simulink model "TailSitter_waypoints_continuous"  (R2018b)
settings: Solver=VariableStepAuto  StartTime=0.0  StopTime=400  RelTol=1e-3
values from neighbouring files (symbols this model uses):
  p =     [ds.mat]    (also in vxs.mat)
undefined symbols (not defined in the file or in its folder): quatnormalize
libraries: aerolibutil x18, simulink x6, sharedutil x3, vrlib x2, simulink_extras x2, sharedtransform x1
(part 4 of 4)

== matlab function TailSitter_waypoints_continuous/TailSitter/tailsittersimv2 ==
  data: omegaLdot output; omegaRdot output; deltaLdot output; deltaRdot output; qdot output; wdot output; vdot output; omegaL input; omegaR input; deltaL input; deltaR input; u_omegaL input; u_omegaR input; u_deltaL input; u_deltaR input; q input; w input; v input; p parameter; alpha output; Beta output; g_out output
function [ omegaLdot, omegaRdot, deltaLdot, deltaRdot, qdot,wdot,vdot, alpha, Beta, g_out] = ...
    tailsitter_v2(omegaL, omegaR, deltaL, deltaR, u_omegaL, u_omegaR, u_deltaL, ...
    u_deltaR, q,w,v, p)

% Set output port dim
omegaLdot = 0;
omegaRdot = 0;
deltaLdot = 0;
deltaRdot = 0;
alpha = 0;
Beta = 0;
qdot = zeros(4,1);
wdot = zeros(3,1);
vdot = zeros(3,1);
g_out = zeros(3,1);

% Map inputs
vx = v(1);
vy = v(2);
vz = v(3);

wx = w(1);
wy = w(2);
wz = w(3);

q0 = q(1);
q1 = q(2);
q2 = q(3);
q3 = q(4);

% function handles not supported, so adding here directly
c = @(y) 0.28 - (0.28-0.09).*abs(y)./(p.b/2); % This should be pretty accurate
% Lift curves
CL = @(alpha) p.CL_A*sin(p.CL_B.*alpha)+p.CL_C; % These are wrong, just placeholders
CD = @(alpha) p.CD_A-p.CD_A.*cos(p.CD_B.*alpha)+p.CD_C;

alpha = atan2(vz,vx);

%Thrust
TL = p.K_T .* omegaL.^2;
TR = p.K_T .* omegaR.^2;

% airflow in thrust wake
v_w_L = p.b_w .* omegaL; %[b_w .* omegaL; vy; vz];
v_w_R = p.b_w .* omegaR;
%alpha_wL = atan2(vz,v_w_L);
%alpha_wR = atan2(vz,v_w_R);

% Quaternion
qdot = 0.5.*[-q1 -q2 -q3; ...
            q0 -q3 q2; ...
            q3 q0 -q1; ...
            -q2 q1 q0]*w;

% inputs
deltaLdot = p.K_deltaL .* (-deltaL + u_deltaL);
deltaRdot = p.K_deltaR .* (-deltaR + u_deltaR);
omegaLdot = p.K_omegaL .* (-omegaL + u_omegaL);
omegaRdot = p.K_omegaR .* (-omegaR + u_omegaR);

% gravity
% To get vector g in bf from wf
% we need to rotate it by q_wf, or conj(q_bf)
qc = quatconj([q0 q1 q2 q3]); %
qc0 = qc(1);
qc1 = qc(2);
qc2 = qc(3);
qc3 = qc(4);
gravity = p.g .* [2.*(qc1.*qc3 + qc0.*qc2); ...
                2.*(qc2.*qc3 - qc0.*qc1); ...
                (qc0.^2 - qc1.^2 - qc2.^2 + qc3.^2);
                zeros(3+4+4,1)];
g_out = gravity(1:3,1);
% Inertial forces
inertialF = -[2*(vz.*wy - vy.*wz); ...
             2*(vx.*wz - vz.*wx); ...
             2*(vy.*wx - vx.*wy); ...
             (p.Iz - p.Iy).*wy.*wz./p.Ix; ...
             (p.Ix - p.Iz).*wx.*wz./p.Iy; ...
             (p.Iy - p.Ix).*wx.*wy./p.Iz; ...
             zeros(8,1)];
%Sideslip
Beta = atan2(vy,vx);

% Winglets
CLB = @(beta) p.CLB_A*sin(p.CLB_B.*beta); % These are wrong, just placeholders
CDB = @(beta) p.CDB_A-p.CDB_A.*cos(p.CDB_B.*beta);
L_W = -p.rho * sqrt(vx.^2+vy.^2) * p.SW * (CLB(Beta)*vx + CDB(Beta)*vy); % Lift in bodyframe, y
D_W = p.rho * sqrt(vx.^2+vy.^2) * p.SW * (-CLB(Beta)*vy + CDB(Beta)*vx); % Drag in bodyfram, x

% MAIN WING
% Lift inside wake
LLT = p.Sw_w * 0.5 * p.rho * abs(v_w_L) .* CL(0).*v_w_L ;
LRT = p.Sw_w * 0.5 * p.rho * abs(v_w_R) .* CL(0).*v_w_R ;
% Lift outside wake
LL = p.Sw * 0.5 * p.rho * sqrt(vx.^2 + vz.^2) .* ...
    (CL(alpha).*vx + CD(alpha).*vz);
LR = LL; % Yeah we -could- combine these, but too late!
% Drag inside wake
DLT = p.Sw_w * 0.5 * p.rho * abs(v_w_L) * CD(0) * v_w_L;
DRT = p.Sw_w * 0.5 * p.rho * abs(v_w_R) * CD(0) * v_w_R;
% Drag outside wake
DL = p.Sw * 0.5 * p.rho * sqrt(vx.^2  + vz.^2) .* ...
    (-CL(alpha).*vz + CD(alpha).*vx);
DR = DL; % Yeah, we -could- combine these as well...

% AILERONS
% Lift inside wake, signs bc rotation dir of aileron
FLT = -p.CLdelta * 0.5*p.rho*v_w_L.^2 * p.Saw * deltaL;
FRT = -p.CLdelta * 0.5*p.rho*v_w_R.^2 * p.Saw * deltaR;
% Lift outside wake
FL = -sign(vx).*p.CLdelta * 0.5*p.rho*(vx.^2 + vy.^2 + vz.^2) * p.Sa * deltaL;
FR = -sign(vx).*p.CLdelta * 0.5*p.rho*(vx.^2 + vy.^2 + vz.^2) * p.Sa * deltaR;
% Drag inside wake
DalphaLT =p.CDdelta * 0.5*p.rho*v_w_L.^2 * p.Saw * abs(deltaL);
DalphaRT = p.CDdelta * 0.5*p.rho*v_w_R.^2 * p.Saw * abs(deltaR);
% Drag outside wake, we add sign of vx because we might be reversing?
DalphaL = sign(vx).*p.CDdelta * 0.5*p.rho*(vx.^2 + vy.^2 + vz.^2) * p.Sa * abs(deltaL);
DalphaR = sign(vx).*p.CDdelta * 0.5*p.rho*(vx.^2 + vy.^2 + vz.^2) * p.Sa * abs(deltaR);

% f1
 % diff in ail deflection
  % inside wake
  % outside wake
 % resmom roll,
 % roll due to yaw rate
 % moment due to sideslip
alphal_rmr = @(y) atan2(vz+wx.*y, vx);
restmomroll = @(y) y .* c(y) .* sqrt(vx.^2 + (vz+wx.*y).^2) .* ...
    (CL(alphal_rmr(y)).*vx + CD(alphal_rmr(y)).*(vz+wx.*y));
alphal_rwz = @(y) atan2(vz, vx-wz.*y);
rollduetowz = @(y) y .* c(y) .* sqrt((vx-wz.*y).^2 + vz.^2) .* ...
    (CL(alphal_rwz(y)).*(vx-wz*y) + CD(alphal_rwz(y)).*vz);
f1 = p.yf.*(FLT+FL -FRT-FR) ...
    -0.5*p.rho.*quadgk(restmomroll,-p.yW,p.yW) ... % between wakes
     -0.5*p.rho.*quadgk(restmomroll,-p.yWEE,-p.yWE) ... % outside left wake
      -0.5*p.rho.*quadgk(restmomroll,p.yWE,p.yWEE) ... % outside right wake
    -0.5*p.rho.*quadgk(rollduetowz,-p.yW,p.yW) ... between wakes
     -0.5*p.rho.*quadgk(rollduetowz,-p.yWEE,-p.yWE) ... left side
      -0.5*p.rho.*quadgk(rollduetowz, p.yWE,p.yWEE) ... right side
    +p.zW*L_W;
% f2
 % joint ail deflection
  % inside wake
  % outside wake
 % pitch moment
 % restmom pitch rate, --- compensate for wake!
 % Pitch from winglets
f2 = p.xf.*(FLT+FL+FRT+FR) ...
    ... %+ 0.5*p.rho*p.Cmyl*(2*p.Sw.*(vx.^2+vy.^2+vz.^2)+p.Sw_w*(v_w_L.^2 + v_w_R.^2) ) ...
    -p.xac.*(LL+LR+LLT+LRT) ... % We do not assume Pith coeff static.
    -wy.*p.rho.*2.*p.Sw.*p.Cwy.*sqrt(vx.^2 + vz.^2) ...
    +p.zW*D_W;
% f3
 % diff in T
 % mom due to sideslip
 % restmom yaw rate, compensate for outside wake
restmomwz = @(y) y .* c(y) .* sqrt((vx-wz.*y).^2 + vz.^2) .* ...
    (-CL(alphal_rwz(y)).*vz + CD(alphal_rwz(y)).*(vx-wz.*y));
f3 = p.yt.*(TL-TR) ...
     -p.xW*L_W ...
     +0.5*quadgk(restmomwz,-p.yW,p.yW) ...
     +0.5*quadgk(restmomwz,-p.yWEE,-p.yWE) ...
     +0.5*quadgk(restmomwz, p.yWE,p.yWEE);
 
%velocities
vxdot = (TL +TR -DL -DR -DLT -DRT -D_W -DalphaL -DalphaR -DalphaLT -DalphaRT)./p.m;
vydot = L_W./p.m;
vzdot = (-LL -LR -LLT -LRT +FL +FR +FLT +FRT)./p.m;

% angular rates
wxdot = f1./p.Ix;
wydot = f2./p.Iy;
wzdot = f3./p.Iz;

%if any(abs(vxdot) > 100)
%    p.m
%end

statesdot = gravity + inertialF +  ...
    [vxdot;vydot;vzdot;wxdot;wydot;wzdot;qdot;...
    deltaLdot;deltaRdot;omegaLdot;omegaRdot];

vdot = statesdot(1:3);
wdot = statesdot(4:6);
qdot = statesdot(7:10);
deltaLdot = statesdot(11);
deltaRdot = statesdot(12);
omegaLdot = statesdot(13);
omegaRdot = statesdot(14);

== matlab function TailSitter_waypoints_continuous/TailSitter/myQuatNorm ==
  data: q input; n output
function n = fcn(q)

n = sqrt(q(1).^2 + q(2).^2 + q(3).^2 + q(4).^2);

== matlab function TailSitter_waypoints_continuous/MATLAB Function ==
  data: u input; y output
function y = norm(u)

y = sqrt(sum(u.^2));

== matlab function TailSitter_waypoints_continuous/TailSitter/MATLAB Function ==
  data: time input; w output
function w = rotsteps(time)

stept = 10;
wt = 10;
reverse = 0;
if time<stept
    w = [0.1,0,0];
elseif time<stept+wt
    if reverse
        w = [-0.1,0,0];
    else
        w = zeros(1,3);
    end
elseif time<2*stept+wt
    w = [0,0,0.1];
elseif time<2*stept+2*wt
    if reverse
        w = [0,0,-0.1];
    else
        w = zeros(1,3);
    end
else
    w = [0,0.1,0];
end

== matlab function TailSitter_waypoints_continuous/MATLAB Function2 ==
  data: q_wf input; q_ref output
function q_ref = refquat(q_wf)

% TODO: Figure out how to set a good reference quaternion.
q_ref = q_wf;

== matlab function TailSitter_waypoints_continuous/MATLAB Function1 ==
  data: v_ref input; q_ref output; u_jointT output
function [q_ref,u_jointT] = ref_quat(v_ref)


q_ref = [1,0,0,0]';
u_jointT = 300;

% We have output of 5dof.
% Input is 3dof.
% We can extend input dof by saying we want wings to be horizontal, now
% total in is 4dof.


%Construct quaterion from several different rotations?

== matlab function TailSitter_waypoints_continuous/linegenerator ==
  settings: updateMethod=DISCRETE
  data: v_wf input; dist2line2d output; r input; altError output; p parameter; thetaerr output; rspeed output; linevec output; vec2line output; wpN output
function [dist2line2d,altError, thetaerr, rspeed, linevec, vec2line, wpN] = LineGenerator(v_wf,r,p)

% Keep track of which waypoint we are going to
persistent waypointno;
persistent wp;
persistent wp_prev;
if isempty(waypointno)
    waypointno = 2;
    wp = p.waypoints(waypointno,:)';
    wp_prev = p.waypoints(waypointno-1,:)';
end

%initialize variables
dist2line2d = 0;
altError = 0;
thetaerr = 0;
rspeed = 0;
vec2line = [0,0,0]';

% if current waypoint is the start wp/home wp jump immediately to next.
if sqrt( sum( (wp(1:3)-r).^2 ) ) <= p.wpradius
    if waypointno < p.numwp
        waypointno = waypointno+1;
    else
        waypointno = 2; % we always skip home wp at origin
    end
    wp_prev = wp;
    wp = p.waypoints(waypointno,:)';
end
rspeed = wp(4);

% find vector between last waypoint and current target
linevec = (wp(1:3)-wp_prev(1:3))./sqrt( sum((wp(1:3)-wp_prev(1:3)).^2) );

% Figure out if goal is ahead of us or if we passed it/missed it.
%if dot(v_wf(1:3), wp(1:3)-r(1:3)) < 0
%    linevec(1:2) = - linevec(1:2);
%end
% THe above doesn't work. lets start discretizing instead

% find angle in x-y plane of vector
thetastar = atan2(linevec(2), linevec(1));
% find our current heading
theta = atan2(v_wf(2),v_wf(1));
% Error in direction along line / be paralell with line
thetaerr = thetastar - theta;


% Find the vector that describes the vector to the closest point on the
% line
a = wp_prev(1:3);
n = linevec;
vec2line = a-r - dot(a-r,n)*n;
altError = vec2line(3);
dist2line2d = sqrt( sum( vec2line(1:2).^2 ));
wpN = waypointno;
